simulink model "Series_Resonant_converter"  (R2024b)
settings: Solver=ode4  StartTime=0.0  StopTime=0.03  FixedStep=1/(1000*35000)  RelTol=1e-3
libraries: spsVoltageMeasurementLib x7, spsSeriesRLCBranchLib x5, spsCurrentMeasurementLib x5, spsDiodeLib x4, spsIGBTDiodeLib x4, spsOnDelayLib x2, spsDCVoltageSourceLib x1, sps_lib x1
settings Model: Creator=adity  LastModifiedBy=adity

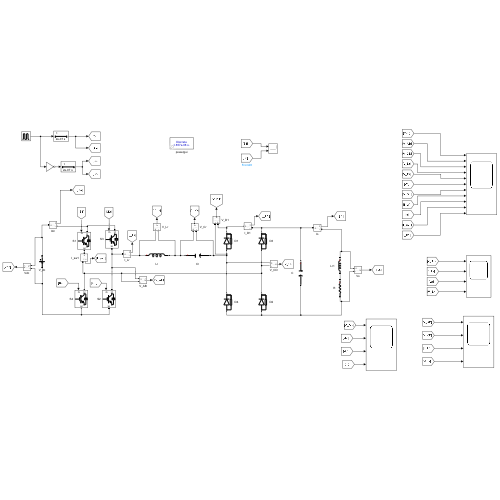
[thumbnail: Simulink's stored preview of the top-level diagram]
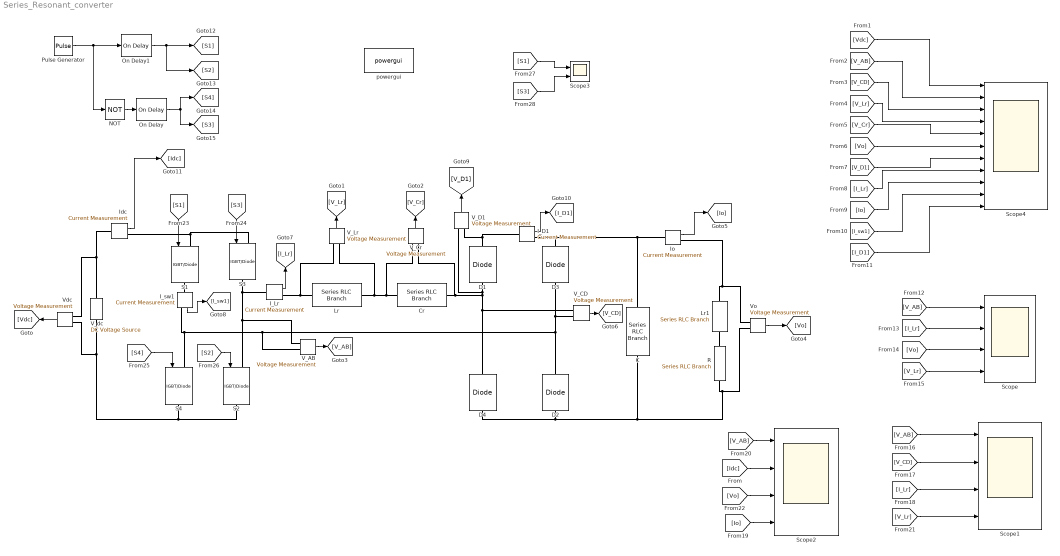
== system Series_Resonant_converter ==
  C : spsSeriesRLCBranchLib/Series RLC Branch  LConnTagsString=__new0  RConnTagsString=__new0  BranchType=C  Resistance=1  Inductance=1e-3  SetiL0=off  InitialCurrent=0  Capacitance=420e-6  Setx0=off  InitialVoltage=0  Measurements=None
  Cr : spsSeriesRLCBranchLib/Series RLC Branch  LConnTagsString=__new0  RConnTagsString=__new0  BranchType=C  Resistance=1  Inductance=1e-3  SetiL0=off  InitialCurrent=0  Capacitance=480.23e-9  Setx0=off  InitialVoltage=0  Measurements=Branch voltage
  D{1..4} (4 alike) : spsDiodeLib/Diode  Ron=1e-2  Lon=0  Vf=0  IC=0  UseSnubber=0  Rs=500  Cs=250e-9  Measurements=off
  I_D1 : spsCurrentMeasurementLib/Current Measurement  PhasorSimulation=off  OutputType=Complex  PSBequivalent=0
  I_Lr : spsCurrentMeasurementLib/Current Measurement  PhasorSimulation=off  OutputType=Complex  PSBequivalent=0
  I_sw1 : spsCurrentMeasurementLib/Current Measurement  PhasorSimulation=off  OutputType=Complex  PSBequivalent=0
  Idc : spsCurrentMeasurementLib/Current Measurement  PhasorSimulation=off  OutputType=Complex  PSBequivalent=0
  Io : spsCurrentMeasurementLib/Current Measurement  PhasorSimulation=off  OutputType=Complex  PSBequivalent=0
  Lr : spsSeriesRLCBranchLib/Series RLC Branch  LConnTagsString=__new0  RConnTagsString=__new0  BranchType=L  Resistance=1  Inductance=84.23e-6  SetiL0=off  InitialCurrent=0  Capacitance=1e-6  Setx0=off  InitialVoltage=0  Measurements=Branch voltage and current
  Lr1 : spsSeriesRLCBranchLib/Series RLC Branch  LConnTagsString=__new0  RConnTagsString=__new0  BranchType=L  Resistance=1  Inductance=1e-6  SetiL0=off  InitialCurrent=0  Capacitance=1e-6  Setx0=off  InitialVoltage=0  Measurements=Branch voltage and current
  NOT : Logic  Operator=NOT  IconShape=distinctive  AllPortsSameDT=off  OutDataTypeStr=boolean
  On Delay : spsOnDelayLib/On Delay  DelayType=On delay  delay=200e-9  ic=0  Ts=0
  On Delay1 : spsOnDelayLib/On Delay  DelayType=On delay  delay=200e-9  ic=0  Ts=0
  Pulse Generator : DiscretePulseGenerator  PulseType=Time based  Period=1/35000  PulseWidth=50
  R : spsSeriesRLCBranchLib/Series RLC Branch  LConnTagsString=__new0  RConnTagsString=__new0  BranchType=R  Resistance=100  Inductance=1e-3  SetiL0=off  InitialCurrent=0  Capacitance=1e-6  Setx0=off  InitialVoltage=0  Measurements=Branch voltage and current
  S{1..4} (4 alike) : spsIGBTDiodeLib/IGBT//Diode  Ron=1e-2  Rs=1e5  Cs=inf  Measurements=off
  Scope : Scope  NumInputPorts=4
  Scope1 : Scope  NumInputPorts=4
  Scope2 : Scope  NumInputPorts=4
  Scope3 : Scope  NumInputPorts=2
  Scope4 : Scope  NumInputPorts=11
  V_AB : spsVoltageMeasurementLib/Voltage Measurement  PhasorSimulation=off  OutputType=Complex  PSBequivalent=0
  V_CD : spsVoltageMeasurementLib/Voltage Measurement  PhasorSimulation=off  OutputType=Complex  PSBequivalent=0
  V_Cr : spsVoltageMeasurementLib/Voltage Measurement  PhasorSimulation=off  OutputType=Complex  PSBequivalent=0
  V_D1 : spsVoltageMeasurementLib/Voltage Measurement  PhasorSimulation=off  OutputType=Complex  PSBequivalent=0
  V_Lr : spsVoltageMeasurementLib/Voltage Measurement  PhasorSimulation=off  OutputType=Complex  PSBequivalent=0
  V_dc : spsDCVoltageSourceLib/DC Voltage Source  Amplitude=20  Measurements=None
  Vdc : spsVoltageMeasurementLib/Voltage Measurement  PhasorSimulation=off  OutputType=Complex  PSBequivalent=0
  Vo : spsVoltageMeasurementLib/Voltage Measurement  PhasorSimulation=off  OutputType=Complex  PSBequivalent=0
  powergui : sps_lib/powergui  Priority=1  SimulationMode=Discrete  SampleTime=1/(1000*35000)  frequency=60  Iterations=50  frequencyindice=0  Pbase=100e6  ErrMax=1e-4  UnitsV=kV  UnitsW=MW  buscounter=0  FunctionMessages=off  echomessages=off  EnableUseOfTLC=off  CurrentSourceSwitches=off  DisableSnubberDevices=off  DisableRonSwitches=off  DisableVfSwitches=off  DisplayEquations=off  AutomaticDiscreteSolvers=off  SolverType=Tustin/Backward Euler (TBE)  Interpol=off  ExternalGateDelay=off  methode=off  Ts=100  x0status=blocks  SPID=on  SwTol=0  HookPort=off  NonlinearTolerance=1e-4  nMaxIteration=100  ContinueOnMaxIteration=off  RestoreLinks=warning  ResistiveCurrentMeasurement=off  Frange=[0:2:500]  Ylog=off  Xlog=on  ShowGrid=off  save=off  variable=ZData  structure=0  ZoomFFT=off  StartTime=0.0  cycles=1  DisplayStyle=1  fundamental=60  FreqAxis=off  MaxFrequency=1000  frequencyindicesteady=1  RmsSteady=1  display=off
  wires:
  NOT/1 -> On Delay/1
  Pulse Generator/1 -> On Delay1/1, NOT/1
  Vdc/1 -> [Vdc]
  V_Lr/1 -> [V_Lr]
  V_Cr/1 -> [V_Cr]
  V_AB/1 -> [V_AB]
  Vo/1 -> [Vo]
  Io/1 -> [Io]
  V_CD/1 -> [V_CD]
  I_Lr/1 -> [I_Lr]
  I_sw1/1 -> [I_sw1]
  V_D1/1 -> [V_D1]
  I_D1/1 -> [I_D1]
  [Vo] -> Scope4/6
  [Vdc] -> Scope4/1
  [V_AB] -> Scope4/2
  [V_CD] -> Scope4/3
  [V_Lr] -> Scope4/4
  [V_Cr] -> Scope4/5
  [I_D1] -> Scope4/11
  [I_sw1] -> Scope4/10
  [Io] -> Scope4/9
  [I_Lr] -> Scope4/8
  [V_D1] -> Scope4/7
  [V_AB] -> Scope/1
  [I_Lr] -> Scope/2
  [Vo] -> Scope/3
  [V_Lr] -> Scope/4
  [V_AB] -> Scope1/1
  [V_CD] -> Scope1/2
  [I_Lr] -> Scope1/3
  [V_Lr] -> Scope1/4
  [V_AB] -> Scope2/1
  [Idc] -> Scope2/2
  Idc/1 -> [Idc]
  [Vo] -> Scope2/3
  [Io] -> Scope2/4
  On Delay/1 -> [S3], [S4]
  On Delay1/1 -> [S2], [S1]
  [S1] -> S1/1
  [S3] -> S3/1
  [S2] -> S2/1
  [S4] -> S4/1
  [S1] -> Scope3/1
  [S3] -> Scope3/2
  connections:
  Vdc/LConn1 -- Idc/LConn1 -- V_dc/RConn1
  S2/RConn1 -- S4/RConn1 -- Vdc/LConn2 -- V_dc/LConn1
  Cr/LConn1 -- V_Cr/LConn1 -- V_Lr/LConn2 -- Lr/RConn1
  D4/RConn1 -- V_Cr/LConn2 -- Cr/RConn1 -- V_D1/LConn2 -- D1/LConn1 -- V_CD/LConn1
  C/LConn1 -- Io/LConn1 -- I_D1/RConn1 -- D3/RConn1
  D4/LConn1 -- Vo/LConn2 -- R/RConn1 -- C/RConn1 -- D2/LConn1
  Lr/LConn1 -- I_Lr/RConn1 -- V_Lr/LConn1
  V_AB/LConn2 -- D3/LConn1 -- V_CD/LConn2 -- D2/RConn1 -- I_sw1/RConn1 -- S4/LConn1
  S3/RConn1 -- I_Lr/LConn1 -- S2/LConn1 -- V_AB/LConn1
  Io/RConn1 -- Vo/LConn1 -- Lr1/LConn1
  I_sw1/LConn1 -- S1/RConn1
  I_D1/LConn1 -- V_D1/LConn1 -- D1/RConn1
  Lr1/RConn1 -- R/LConn1
  S3/LConn1 -- Idc/RConn1 -- S1/LConn1
